simulink model "SystemIdentification"  (R2022a)
settings: Solver=ode1  StartTime=0.0  StopTime=20  FixedStep=0.1  RelTol=1e-3
libraries: dspsrcs4 x3
settings Model: Creator=Jan-Robin  LastModifiedBy=Jan-Robin

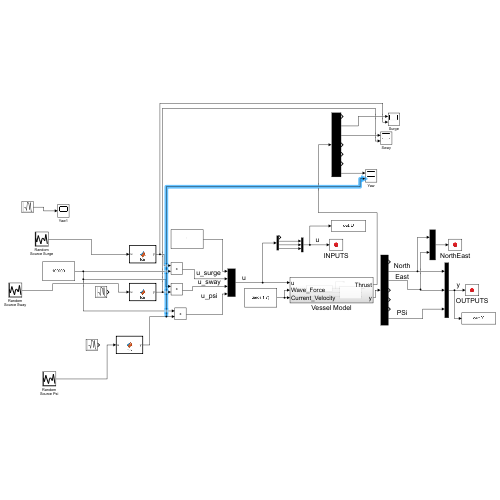
[thumbnail: Simulink's stored preview of the top-level diagram]
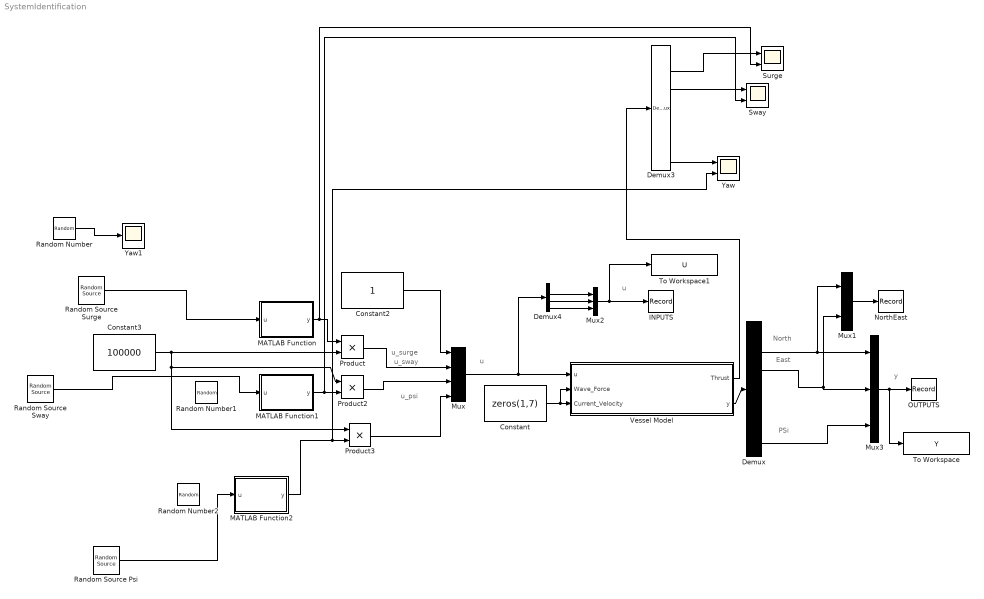
== system SystemIdentification ==
  note: u_sway
  note: y
  note: PSi
  note: u
  note: u_surge
  note: East
  note: North
  note: u
  note: u_psi
  Constant : Constant  Value=zeros(1,7)
  Constant2 : Constant
  Constant3 : Constant  Value=100000
  Demux : Demux  Outputs=7
  Demux3 : Demux  Outputs=7
  Demux4 : Demux
  INPUTS : Record  VariableName=INPUT  RecordToWorkspace=on  FileSettingsInternal="{\"entries\":[{\"content\":{\"excelSettings\":{\"content\":{},\"type\":\"Streamout.ExcelSettings\"}},\"type\":\"Streamout.FileSettingStorage\",\"uuid\":\"\"}],\"packageUris\":[\"http:\\/\\/schema.mathworks.com\\/mf0\\/streamout_blocks\\/R2020a\"],\"version\":\"1.0\"}"  SignalsInternal="{\"entries\":[{\"content\":{\"signals\":[{\"content\":{\"blockPath\":[],\"channel\":[],\"dimensions\":[3],\"domain\":\"\",\"hasChildren\":true,\"lineColor\":\"#b746ff\",\"plots\":[],\"port\":1,\"sid\":[\"\"],\"signalID\":351,\"signalName\":\"Mux2\"},\"type\":\"RecordBlkView.Signal\",\"uuid\":\"\"},{\"content\":{\"blockPath\":[],\"channel\":[1],\"dimensions\":[3],\"domain\":\"\",\"lineColor\":\"#4dbeee\",\"parentID\":351,\"plots\":[1],\"port\":1,\"sid\":[\"\"],\"signalID\":352,\"signalName\":\"Mux2\"},\"type\":\"RecordBlkView.Signal\",\"uuid\":\"\"},{\"content\":{\"blockPath\":[],\"channel\":[2],\"dimensions\":[3],\"domain\":\"\",\"lineColor\":\"#0072bd\",\"parentID\":351,\"plots\":[1],\"port\":1,\"sid\":[\"\"],\"signalID\":391,\"signalName\":\"Mux2\"},\"type\":\"RecordBlkView.Signal\",\"uuid\":\"\"},{\"content\":{\"blockPath\":[],\"channel\":[3],\"dimensions\":[3],\"domain\":\"\",\"lineColor\":\"#d95319\",\"parentID\":351,\"plots\":[1],\"port\":1,\"sid\":[\"\"],\"signalID\":392,\"signalName\":\"Mux2\"},\"type\":\"RecordBlkView.Signal\",\"uuid\":\"\"}]},\"type\":\"RecordBlkView.InputSignals\",\"uuid\":\"\"}],\"packageUris\":[\"http:\\/\\/schema.mathworks.com\\/mf0\\/streamout_blocks\\/R2020a\"],\"version\":\"1.0\"}"  VisualizationBindings="{\"sparklinesplugin\":{\"info\":[{\"bindingParametersList\":[],\"subplotID\":1}]}}"
  MATLAB Function : MATLAB Function  TreatAsAtomicUnit=on
  MATLAB Function1 : MATLAB Function  TreatAsAtomicUnit=on
  MATLAB Function2 : MATLAB Function  TreatAsAtomicUnit=on
  Mux : Mux
  Mux1 : Mux  Inputs=2
  Mux2 : Mux  Inputs=3
  Mux3 : Mux  Inputs=3
  NorthEast : Record  VariableName=xydata  Filename=C:\Users\Jan-Robin\OneDrive - Troms og Finnmark fylkeskommune\Documents\Studie\Master\OSP\data.xlsx  RecordToWorkspace=on  RecordToFile=on  FileSettingsInternal="{\"entries\":[{\"content\":{\"excelSettings\":{\"content\":{},\"type\":\"Streamout.ExcelSettings\"}},\"type\":\"Streamout.FileSettingStorage\",\"uuid\":\"\"}],\"packageUris\":[\"http:\\/\\/schema.mathworks.com\\/mf0\\/streamout_blocks\\/R2020a\"],\"version\":\"1.0\"}"  Layout=[1 1]  SignalsInternal="{\"entries\":[{\"content\":{\"signals\":[{\"content\":{\"blockPath\":[],\"channel\":[],\"dimensions\":[2],\"domain\":\"\",\"hasChildren\":true,\"lineColor\":\"#ff13a6\",\"plots\":[],\"port\":1,\"sid\":[\"\"],\"signalID\":356,\"signalName\":\"Mux1\"},\"type\":\"RecordBlkView.Signal\",\"uuid\":\"\"},{\"content\":{\"blockPath\":[],\"channel\":[1],\"dimensions\":[2],\"domain\":\"\",\"lineColor\":\"#ff6929\",\"parentID\":356,\"plots\":[],\"port\":1,\"sid\":[\"\"],\"signalID\":357,\"signalName\":\"Mux1\"},\"type\":\"RecordBlkView.Signal\",\"uuid\":\"\"},{\"content\":{\"blockPath\":[],\"channel\":[2],\"dimensions\":[2],\"domain\":\"\",\"lineColor\":\"#139fff\",\"parentID\":356,\"plots\":[],\"port\":1,\"sid\":[\"\"],\"signalID\":393,\"signalName\":\"Mux1\"},\"type\":\"RecordBlkView.Signal\",\"uuid\":\"\"}]},\"type\":\"RecordBlkView.InputSignals\",\"uuid\":\"\"}],\"packageUris\":[\"http:\\/\\/schema.mathworks.com\\/mf0\\/streamout_blocks\\/R2020a\"],\"version\":\"1.0\"}"  VisualizationBindings="{\"sparklinesplugin\":{\"info\":[{\"bindingParametersList\":[],\"subplotID\":1}]}}"
  OUTPUTS : Record  VariableName=OUTPUT  RecordToWorkspace=on  FileSettingsInternal="{\"entries\":[{\"content\":{\"excelSettings\":{\"content\":{},\"type\":\"Streamout.ExcelSettings\"}},\"type\":\"Streamout.FileSettingStorage\",\"uuid\":\"\"}],\"packageUris\":[\"http:\\/\\/schema.mathworks.com\\/mf0\\/streamout_blocks\\/R2020a\"],\"version\":\"1.0\"}"  Layout=[1 1]  SignalsInternal="{\"entries\":[{\"content\":{\"signals\":[{\"content\":{\"blockPath\":[],\"channel\":[],\"dimensions\":[3],\"domain\":\"\",\"hasChildren\":true,\"lineColor\":\"#22b573\",\"plots\":[],\"port\":1,\"sid\":[\"\"],\"signalID\":361,\"signalName\":\"Mux3\"},\"type\":\"RecordBlkView.Signal\",\"uuid\":\"\"},{\"content\":{\"blockPath\":[],\"channel\":[1],\"dimensions\":[3],\"domain\":\"\",\"lineColor\":\"#64d413\",\"parentID\":361,\"plots\":[],\"port\":1,\"sid\":[\"\"],\"signalID\":362,\"signalName\":\"Mux3\"},\"type\":\"RecordBlkView.Signal\",\"uuid\":\"\"},{\"content\":{\"blockPath\":[],\"channel\":[2],\"dimensions\":[3],\"domain\":\"\",\"lineColor\":\"#ff6929\",\"parentID\":361,\"plots\":[],\"port\":1,\"sid\":[\"\"],\"signalID\":394,\"signalName\":\"Mux3\"},\"type\":\"RecordBlkView.Signal\",\"uuid\":\"\"},{\"content\":{\"blockPath\":[],\"channel\":[3],\"dimensions\":[3],\"domain\":\"\",\"lineColor\":\"#b746ff\",\"parentID\":361,\"plots\":[],\"port\":1,\"sid\":[\"\"],\"signalID\":395,\"signalName\":\"Mux3\"},\"type\":\"RecordBlkView.Signal\",\"uuid\":\"\"}]},\"type\":\"RecordBlkView.InputSignals\",\"uuid\":\"\"}],\"packageUris\":[\"http:\\/\\/schema.mathworks.com\\/mf0\\/streamout_blocks\\/R2020a\"],\"version\":\"1.0\"}"  VisualizationBindings="{\"sparklinesplugin\":{\"info\":[{\"bindingParametersList\":[],\"subplotID\":1}]}}"
  Product : Product
  Product2 : Product
  Product3 : Product
  Random Number : RandomNumber  Variance=0.5  Seed=1  SampleTime=1
  Random Number1 : RandomNumber  Variance=0.5  Seed=2  SampleTime=1
  Random Number2 : RandomNumber  Variance=0.5  Seed=3  SampleTime=1
  Random Source Psi : dspsrcs4/Random Source  SrcType=Uniform  NormMethod=Ziggurat  CltLength=12  MinVal=-1  MaxVal=1  MeanVal=0  VarVal=1  RepMode=Not repeatable  rawSeed=1  IsInherit=off  SampMode=Continuous  SampTime=10  SampFrame=1  DataType=Single  OutComplex=Real  OutputFrames=off
  Random Source Surge : dspsrcs4/Random Source  SrcType=Uniform  NormMethod=Ziggurat  CltLength=12  MinVal=-1  MaxVal=1  MeanVal=0  VarVal=1  RepMode=Not repeatable  rawSeed=1  IsInherit=off  SampMode=Continuous  SampTime=10  SampFrame=1  DataType=Single  OutComplex=Real  OutputFrames=off
  Random Source Sway : dspsrcs4/Random Source  SrcType=Uniform  NormMethod=Ziggurat  CltLength=12  MinVal=-1  MaxVal=1  MeanVal=0  VarVal=1  RepMode=Not repeatable  rawSeed=1  IsInherit=off  SampMode=Continuous  SampTime=10  SampFrame=1  DataType=Single  OutComplex=Real  OutputFrames=off
  Surge : Scope  NumInputPorts=2
  Sway : Scope  NumInputPorts=2
  To Workspace : ToWorkspace  VariableName=Y  SampleTime=0.2
  To Workspace1 : ToWorkspace  VariableName=U  SampleTime=0.2
  Vessel Model : Subsystem
  Yaw : Scope  NumInputPorts=2
  Yaw1 : Scope
  wires:
  Mux3/1 -> To Workspace/1, OUTPUTS/1
  Vessel Model/2(y) -> Demux/1
  Mux/1 -> Demux4/1, Vessel Model/1(u)
  Demux4/2 -> Mux2/1
  Demux4/3 -> Mux2/2
  Constant/1 -> Vessel Model/3(Current_Velocity), Vessel Model/2(Wave_Force)
  Demux/2 -> Mux3/1, Mux1/1
  Demux4/4 -> Mux2/3
  Mux1/1 -> NorthEast/1
  Demux/7 -> Mux3/3
  Demux/3 -> Mux3/2, Mux1/2
  Mux2/1 -> To Workspace1/1, INPUTS/1
  MATLAB Function2/1(y) -> Product3/2, Yaw/2
  MATLAB Function1/1(y) -> Product2/2, Sway/2
  Constant3/1 -> Product/2, Product3/1, Product2/1
  Product/1 -> Mux/2
  Constant2/1 -> Mux/1
  Product3/1 -> Mux/4
  Product2/1 -> Mux/3
  Demux3/7 -> Yaw/1
  Demux3/2 -> Surge/1
  MATLAB Function/1(y) -> Surge/2, Product/1
  Demux3/3 -> Sway/1
  Vessel Model/1(Thrust) -> Demux3/1
  Random Number/1 -> Yaw1/1
  Random Source Surge/1 -> MATLAB Function/1(u)
  Random Source Sway/1 -> MATLAB Function1/1(u)
  Random Source Psi/1 -> MATLAB Function2/1(u)

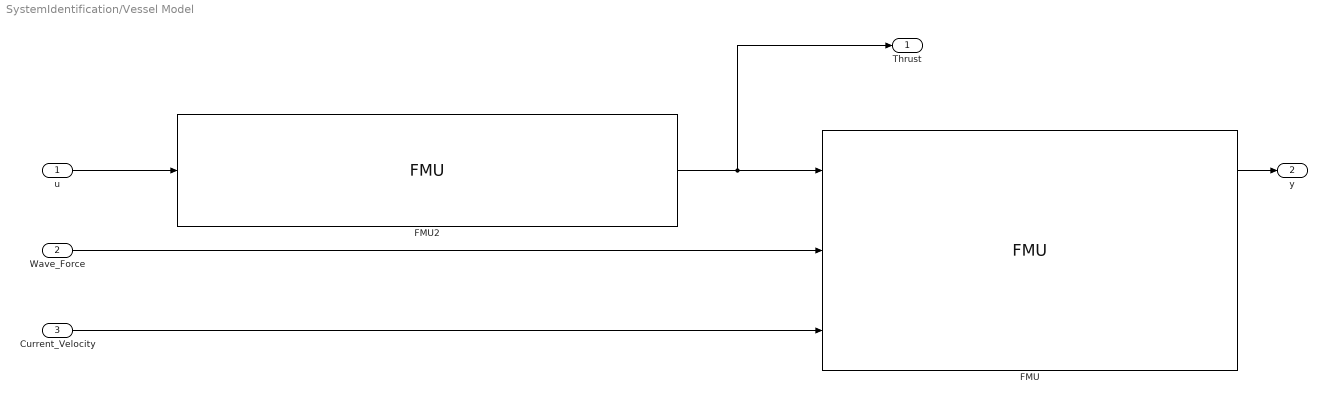
== system SystemIdentification/Vessel Model ==
  u : Inport
  Wave_Force : Inport  Port=2
  Current_Velocity : Inport  Port=3
  FMU : FMU  FMUName=VesselModel.fmu  FMUMode=CoSimulation  Axc=106.0  Ayc=419.0  Bv_0_=44000.0  Bv_1_=0.0  Bv_2_=0.0  Bv_3_=0.0  Bv_4_=0.0  Bv_5_=0.0  Bv_6_=0.0  Bv_7_=177000.0  Bv_8_=0.0  Bv_9_=0.0  Bv_10_=0.0  Bv_11_=0.0  Bv_12_=0.0  Bv_13_=0.0  Bv_14_=0.0  Bv_15_=0.0  Bv_16_=0.0  Bv_17_=0.0  Bv_18_=0.0  Bv_19_=0.0  Bv_20_=0.0  Bv_21_=686000.0  Bv_22_=0.0  Bv_23_=0.0  Bv_24_=0.0  Bv_25_=0.0  Bv_26_=0.0  Bv_27_=0.0  Bv_28_=0.0  Bv_29_=0.0  Bv_30_=0.0  Bv_31_=0.0  Bv_32_=0.0  Bv_33_=0.0  Bv_34_=0.0  Bv_35_=1.0259E+7  Cx=1.0  Cy=0.7812  Dp_0_=5300.0  Dp_1_=0.0  Dp_2_=0.0  Dp_3_=0.0  Dp_4_=0.0  Dp_5_=0.0  Dp_6_=0.0  Dp_7_=21100.0  Dp_8_=0.0  Dp_9_=-20300.0  Dp_10_=0.0  Dp_11_=294000.0  Dp_12_=0.0  Dp_13_=0.0  Dp_14_=1900.0  Dp_15_=0.0  Dp_16_=-68400.0  Dp_17_=0.0  Dp_18_=0.0  Dp_19_=-20300.0  Dp_20_=0.0  Dp_21_=7600.0  Dp_22_=0.0  Dp_23_=-201300.0  Dp_24_=0.0  Dp_25_=0.0  Dp_26_=-68400.0  Dp_27_=0.0  Dp_28_=819700.0  Dp_29_=0.0  Dp_30_=0.0  Dp_31_=294000.0  Dp_32_=0.0  Dp_33_=-201300.0  Dp_34_=0.0  Dp_35_=1.8944E+6  G_0_=0.0  G_1_=0.0  G_2_=0.0  G_3_=0.0  G_4_=0.0  G_5_=0.0  G_6_=0.0  G_7_=0.0  G_8_=0.0  G_9_=0.0  G_10_=0.0  G_11_=0.0  G_12_=0.0  G_13_=0.0  G_14_=2.44E+6  G_15_=0.0  G_16_=1.78E+6  G_17_=0.0  G_18_=0.0  G_19_=0.0  G_20_=0.0  G_21_=5.11E+6  G_22_=0.0  G_23_=0.0  G_24_=0.0  G_25_=0.0  G_26_=1.78E+6  G_27_=0.0  G_28_=1.2737E+8  G_29_=0.0  G_30_=0.0  G_31_=0.0  G_32_=0.0  G_33_=0.0  G_34_=0.0  G_35_=0.0  Lpp=28.9  Minv_0_=1.268E-6  Minv_1_=0.0  Minv_2_=0.0  Minv_3_=0.0  Minv_4_=0.0  Minv_5_=0.0  Minv_6_=0.0  Minv_7_=1.083E-6  Minv_8_=0.0  Minv_9_=1.2E-8  Minv_10_=0.0  Minv_11_=1.0E-9  Minv_12_=0.0  Minv_13_=0.0  Minv_14_=5.9200000000000011E-7  Minv_15_=0.0  Minv_16_=-1.3E-8  Minv_17_=0.0  Minv_18_=0.0  Minv_19_=1.2E-8  Minv_20_=0.0  Minv_21_=1.0000000000000001E-7  Minv_22_=0.0  Minv_23_=-1.0E-9  Minv_24_=0.0  Minv_25_=0.0  Minv_26_=-1.3E-8  Minv_27_=0.0  Minv_28_=1.2E-8  Minv_29_=0.0  Minv_30_=0.0  Minv_31_=1.0E-9  Minv_32_=0.0  Minv_33_=-1.0E-9  Minv_34_=0.0  Minv_35_=2.0E-8  N=20.0  X_DOF_DP_model_Integrator1__InitialCondition_0_=0.0  X_DOF_DP_model_Integrator1__InitialCondition_1_=0.0  X_DOF_DP_model_Integrator1__InitialCondition_2_=0.0  X_DOF_DP_model_Integrator1__InitialCondition_3_=0.0  X_DOF_DP_model_Integrator1__InitialCondition_4_=0.0  X_DOF_DP_model_Integrator1__InitialCondition_5_=0.0  X_DOF_DP_model_Integrator2_InitialCondition_0_=0.0  X_DOF_DP_model_Integrator2_InitialCondition_1_=0.0  X_DOF_DP_model_Integrator2_InitialCondition_2_=0.0  X_DOF_DP_model_Integrator2_InitialCondition_3_=0.0  X_DOF_DP_model_Integrator2_InitialCondition_4_=0.0  X_DOF_DP_model_Integrator2_InitialCondition_5_=0.0  X_DOF_DP_model_Rotate_yaw_T_Constant_Value=0.0  X_DOF_DP_model_Rotate_yaw_T_psi_Value=0.0  X_DOF_DP_model_X_DOF_transformation_Euler_angles_to_att=0.0  X_DOF_DP_model_X_DOF_transformation_Euler_angles_to_att_2=1.0  X_DOF_DP_model_zero_Value=0.0  rho=1025.0  mask(VesselModel [Co-Simulation, v2.0]){}
      mask Display:
      | disp('VesselModel');
      | port_label('output',1,'Vessel_Position');
      | port_label('output',2,'Vessel_Velocity');
      | port_label('output',3,'Vessel_Acceleration');
      | port_label('input',1,'Thrust');
      | port_label('input',2,'Wave_Forces');
      | port_label('input',3,'Current_Velocity');
  FMU2 : FMU  FMUName=ThrusterDynamics.fmu  FMUMode=CoSimulation  Heave_Thrust=struct('Value',0.0)  Merge1=struct('InitialOutput',0.0)  Pitch_Thrust=struct('Value',0.0)  Roll_Thrust=struct('Value',0.0)  Thruster_Dynamics=struct('Surge_Thrust_Dynamics',struct('A',-0.2,'C',0.2),'Sway_Thrust_Dynamics',struct('A',-0.2,'C',0.2),'Yaw_Thrust_Dynamics',struct('A',-0.2,'C',0.2))  enableDynamics=on  enableSaturation=on  maxThrust=[1.0E+10,1.0E+10,1.0E+11]  mask(ThrusterDynamics [Co-Simulation, v2.0]){}
      mask Display:
      | disp('ThrusterDynamics');
      | port_label('output',1,'Thrust');
      | port_label('input',1,'Commanded_Thrust');
  Thrust : Outport
  y : Outport  Port=2
  wires:
  u/1 -> FMU2/1
  FMU2/1 -> Thrust/1, FMU/1
  FMU/1 -> y/1
  Wave_Force/1 -> FMU/2
  Current_Velocity/1 -> FMU/3

== matlab function SystemIdentification/MATLAB Function ==
  data: u input; y output
function y = fcn(u)

if (u> 0)
    y=1;

else
    y=-1;
end

== matlab function SystemIdentification/MATLAB Function2 ==
  data: u input; y output
function y = fcn(u)

if (u> 0)
    y=1;

else
    y=-1;
end

== matlab function SystemIdentification/MATLAB Function1 ==
  data: u input; y output
function y = fcn(u)

if (u> 0)
    y=1;

else
    y=-1;
end
